simulink model "LQR_Control_with_Integral"  (R2020a)
settings: Solver=VariableStepAuto  StartTime=0.0  StopTime=5  RelTol=1e-3
values from neighbouring files (symbols this model uses):
  A = [0 1 0 0 ... (first row only)    [LQR_Pendulum.m]
  B = [0; -I_1*C_1/Z; 0; -C_1*I_2/Z]    [LQR_Pendulum.m]
undefined symbols (not defined in the file or in its folder): K
settings Model: Creator=sabir  LastModifiedBy=sabir

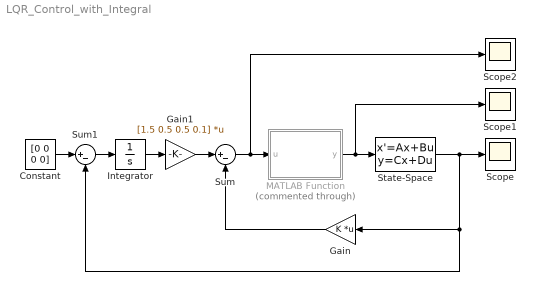
== system LQR_Control_with_Integral ==
  Constant : Constant  Value=[0 0 0 0]
  Gain : Gain  Gain=K  Multiplication=Matrix(K*u)
  Gain1 : Gain  Gain=[1.5 0.5 0.5 0.1]  Multiplication=Matrix(K*u)
  Integrator : Integrator
  MATLAB Function : MATLAB Function  Commented=through  TreatAsAtomicUnit=on
  Scope : Scope
  Scope1 : Scope
  Scope2 : Scope
  State-Space : StateSpace  A=A  B=B  C=eye(4)  D=zeros(4,1)  InitialCondition=[0.25;0.5;0.50;0.1]
  Sum : Sum  Inputs=|+-
  Sum1 : Sum  Inputs=|+-
  wires:
  Integrator/1 -> Gain1/1
  Gain1/1 -> Sum/1
  Sum1/1 -> Integrator/1
  Gain/1 -> Sum/2
  Sum/1 -> Scope2/1, MATLAB Function/1(u)
  Constant/1 -> Sum1/1
  MATLAB Function/1(y) -> Scope1/1, State-Space/1
  State-Space/1 -> Scope/1, Gain/1, Sum1/2

== matlab function LQR_Control_with_Integral/MATLAB Function ==
  data: u input; y output
function y = fcn(u)
if u<3.5 && u>-3.5
    u=0;
end

if u>15
    u=15;
elseif u<-15
    u=-15;
end

y = u;
